simulink model "sender_task"  (Simulink 3.00)
libraries: genlib x2, mathlib x2, speclib x1

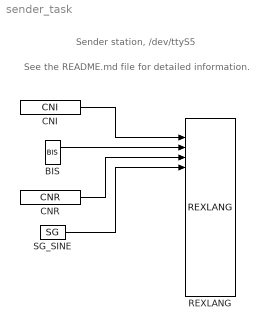
== system sender_task ==
  note: See the README.md file for detailed information.
  note: Sender station, /dev/ttyS5
  BIS : genlib/BIS  Y0=off  t1=1  t2=2  t3=0  t4=4  t5=5  t6=6  t7=7  t8=8  RPT=on
  CNI : mathlib/CNI  icn=87654321
  CNR : mathlib/CNR  ycn=-247.18
  REXLANG : speclib/REXLANG  srcname=sender_rexlang.c  srctype=1: STL  stack=0  debug=1: No check  fname=/dev/ttyS5
  SG_SINE : genlib/SG  isig=1: SINE  amp=10  freq=0.03  phase=0  ifrunit=1: Hz  iphunit=1: degrees
  wires:
  BIS/1 -> REXLANG/3
  CNI/1 -> REXLANG/2
  CNR/1 -> REXLANG/4
  SG_SINE/1 -> REXLANG/5
